simulink model "lab2"  (R2020b)
settings: Solver=VariableStepAuto  StartTime=0.0  StopTime=10.0  RelTol=1e-3
model workspace (MAT data in the model file):
  K1 = Simulink.Parameter
  K1.Value = 50
  K1.DataType = 'auto'
  K1.Dimensions = [1 1]
  K12 = Simulink.Parameter
  K12.Value = 20
  K12.DataType = 'auto'
  K12.Dimensions = [1 1]
  M1 = Simulink.Parameter
  M1.Value = 100
  M1.DataType = 'auto'
  M1.Dimensions = [1 1]
  M2 = Simulink.Parameter
  M2.Value = 20
  M2.DataType = 'auto'
  M2.Dimensions = [1 1]
  b = Simulink.Parameter
  b.Value = 50
  b.DataType = 'auto'
  b.Dimensions = [1 1]
settings Model: Creator=karth  LastModifiedBy=karth

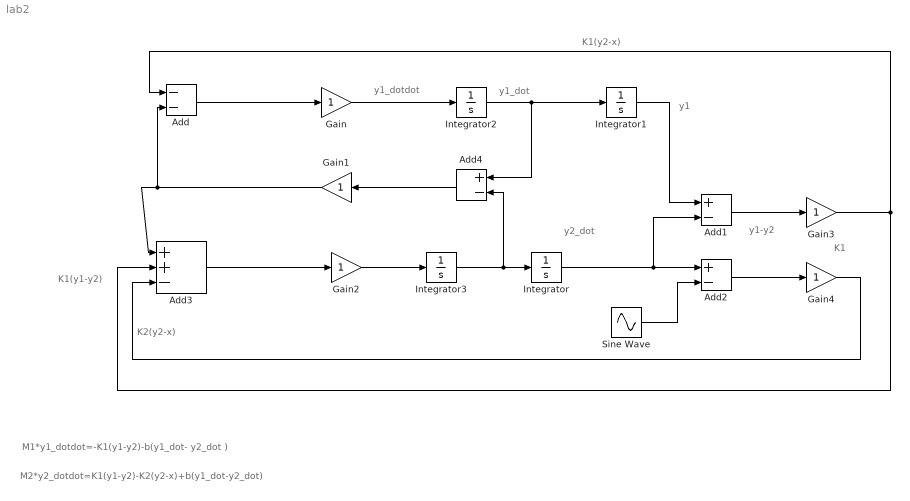
== system lab2 ==
  note: M2*y2_dotdot=K1(y1-y2)-K2(y2-x)+b(y1_dot-y2_dot)
  note: M1*y1_dotdot=-K1(y1-y2)-b(y1_dot- y2_dot )
  note: y1_dotdot
  note: K1(y1-y2)
  note: y2_dot
  note: y1
  note: y1-y2
  note: K1
  note: K2(y2-x)
  note: K1(y2-x)
  note: y1_dot
  Add : Sum  Inputs=--
  Add1 : Sum  Inputs=+-
  Add2 : Sum  Inputs=+-
  Add3 : Sum  Inputs=++-
  Add4 : Sum  Inputs=+-
  Gain{,1..4} (5 alike) : Gain
  Integrator{,1..3} (4 alike) : Integrator
  Sine Wave : Sin  Amplitude=2*pi*100  SampleTime=0
  wires:
  Add/1 -> Gain/1
  Gain/1 -> Integrator2/1
  Integrator2/1 -> Add4/1, Integrator1/1
  Integrator1/1 -> Add1/1
  Add4/1 -> Gain1/1
  Gain1/1 -> Add/2, Add3/1
  Add3/1 -> Gain2/1
  Gain2/1 -> Integrator3/1
  Sine Wave/1 -> Add2/2
  Integrator/1 -> Add1/2, Add2/1
  Add2/1 -> Gain4/1
  Add1/1 -> Gain3/1
  Gain3/1 -> Add3/2, Add/1
  Gain4/1 -> Add3/3
  Integrator3/1 -> Add4/2, Integrator/1
